simulink model "s1"  (R2022a)
settings: Solver=ode1  StartTime=0.0  StopTime=Tsin  FixedStep=0.01  RelTol=1e-3
values from neighbouring files (symbols this model uses):
  alpha1 = x1    [HHmododeslizante2.m]
  amp = 1    [HHmododeslizante2.m]
  beta1 = x2    [HHmododeslizante2.m]
  k5 = 0.3    [HHmododeslizante2.m]
  Lambda = x3    [HHmododeslizante2.m]
libraries: simulink x2
settings Model: Creator=L03037425  LastModifiedBy=danie
settings ModelReferenceCC: EnableRefExpFcnMdlSchedulingChecks=off
settings RTWCC: Description=Generic Real-Time Target

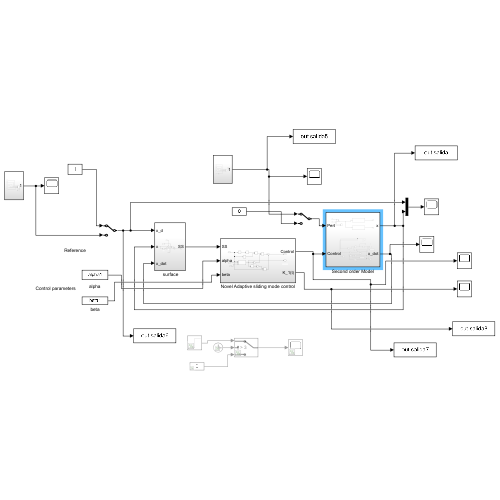
[thumbnail: Simulink's stored preview of the top-level diagram]
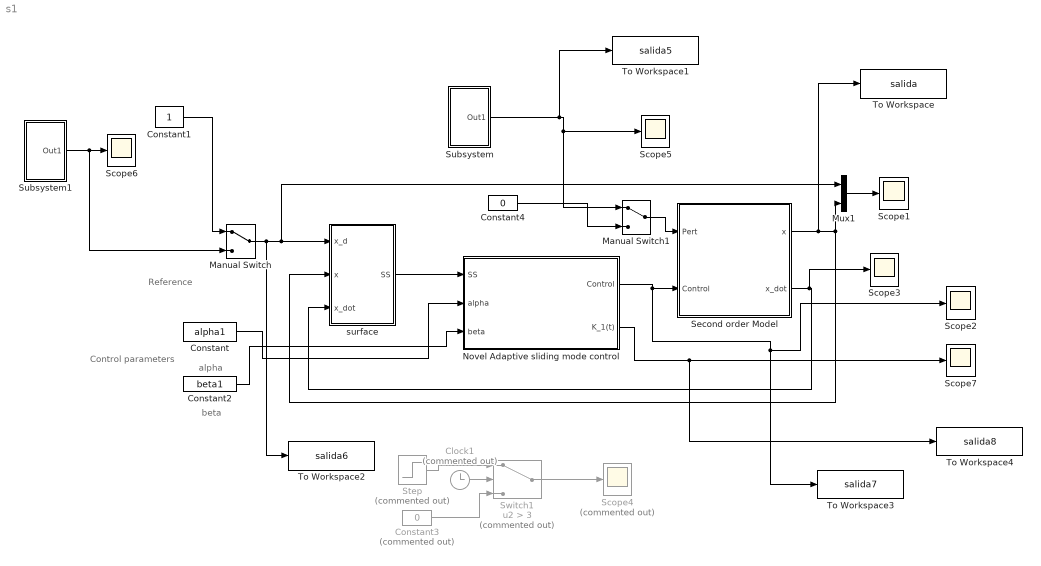
== system s1 ==
  note: Control parameters
  note: beta
  note: alpha
  note: Reference
  " surface" : Subsystem
  Clock1 : Clock  Commented=on
  Constant : Constant  Value=alpha1
  Constant1 : Constant
  Constant2 : Constant  Value=beta1
  Constant3 : Constant  Commented=on  Value=0
  Constant4 : Constant  Value=0
  Manual Switch : ManualSwitch
  Manual Switch1 : ManualSwitch
  Mux1 : Mux  Inputs=2
  Novel Adaptive sliding mode control : Subsystem
  Scope{1..3,5..7} (6 alike) : Scope
  Scope4 : Scope  Commented=on
  Second order Model : Subsystem
  Step : Step  Commented=on  Time=5  SampleTime=0
  Subsystem : Subsystem
  Subsystem1 : Subsystem
  Switch1 : Switch  Commented=on  Criteria=u2 > Threshold  Threshold=3  SaturateOnIntegerOverflow=off  InputSameDT=off
  To Workspace : ToWorkspace  VariableName=salida  SampleTime=-1
  To Workspace1 : ToWorkspace  VariableName=salida5  SampleTime=-1
  To Workspace2 : ToWorkspace  VariableName=salida6  SampleTime=-1
  To Workspace3 : ToWorkspace  VariableName=salida7  SampleTime=-1
  To Workspace4 : ToWorkspace  VariableName=salida8  SampleTime=-1
  wires:
  Constant1/1 -> Manual Switch/1
  " surface"/1(SS) -> Novel Adaptive sliding mode control/1(SS)
  Novel Adaptive sliding mode control/1(Control) -> To Workspace3/1, Scope2/1, Second order Model/2(Control)
  Manual Switch/1 -> To Workspace2/1, Mux1/1, " surface"/1(x_d)
  Second order Model/2(x_dot) -> Scope3/1, " surface"/3(x_dot)
  Second order Model/1(x) -> To Workspace/1, " surface"/2(x), Mux1/2
  Novel Adaptive sliding mode control/2(K_1(t)) -> To Workspace4/1, Scope7/1
  Constant/1 -> Novel Adaptive sliding mode control/2(alpha)
  Constant2/1 -> Novel Adaptive sliding mode control/3(beta)
  Mux1/1 -> Scope1/1
  Manual Switch1/1 -> Second order Model/1(Pert)
  Step/1 -> Switch1/1
  Switch1/1 -> Scope4/1
  Clock1/1 -> Switch1/2
  Constant3/1 -> Switch1/3
  Constant4/1 -> Manual Switch1/2
  Subsystem/1(Out1) -> To Workspace1/1, Manual Switch1/1, Scope5/1
  Subsystem1/1(Out1) -> Manual Switch/2, Scope6/1

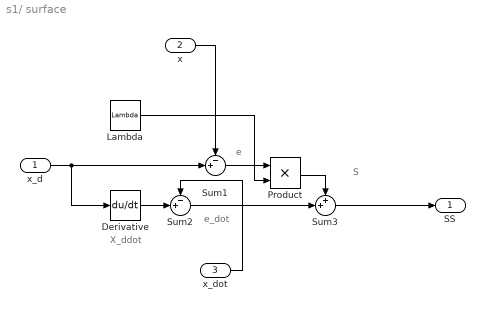
== system s1/ surface ==
  note: S
  note: e_dot
  note: e
  note: X_ddot
  x_d : Inport
  x : Inport  Port=2
  x_dot : Inport  Port=3
  Derivative : Derivative
  Lambda : Constant  Value=Lambda
  Product : Product
  Sum1 : Sum  Inputs=-+|
  Sum2 : Sum  Inputs=-+|
  Sum3 : Sum  Inputs=++|
  SS : Outport
  wires:
  Product/1 -> Sum3/1
  Sum2/1 -> Sum3/2
  x_d/1 -> Derivative/1, Sum1/2
  Lambda/1 -> Product/2
  Derivative/1 -> Sum2/2
  Sum1/1 -> Product/1
  Sum3/1 -> SS/1
  x/1 -> Sum1/1
  x_dot/1 -> Sum2/1

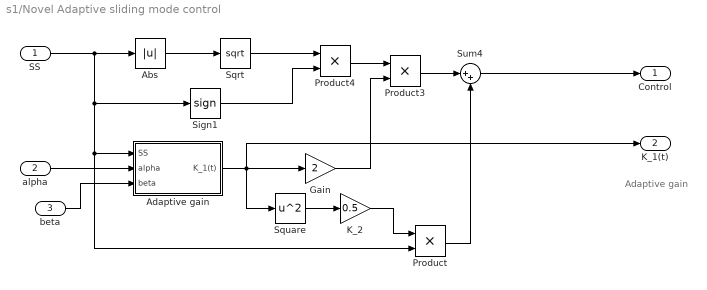
== system s1/Novel Adaptive sliding mode control ==
  note: Adaptive gain
  SS : Inport
  alpha : Inport  Port=2
  beta : Inport  Port=3
  Abs : Abs  SaturateOnIntegerOverflow=off
  Adaptive gain : Subsystem
  Gain : Gain  Gain=2
  K_2 : Gain  Gain=0.5
  Product : Product
  Product3 : Product
  Product4 : Product
  Sign1 : Signum
  Sqrt : Sqrt
  Square : Math  Operator=square
  Sum4 : Sum  Inputs=|++
  Control : Outport
  K_1(t) : Outport  Port=2
  wires:
  SS/1 -> Product/2, Adaptive gain/1(SS), Sign1/1, Abs/1
  Sqrt/1 -> Product4/1
  Product3/1 -> Sum4/1
  Abs/1 -> Sqrt/1
  Product4/1 -> Product3/1
  Sign1/1 -> Product4/2
  Sum4/1 -> Control/1
  Gain/1 -> Product3/2
  Adaptive gain/1(K_1(t)) -> K_1(t)/1, Gain/1, Square/1
  Product/1 -> Sum4/2
  K_2/1 -> Product/1
  Square/1 -> K_2/1
  alpha/1 -> Adaptive gain/2(alpha)
  beta/1 -> Adaptive gain/3(beta)

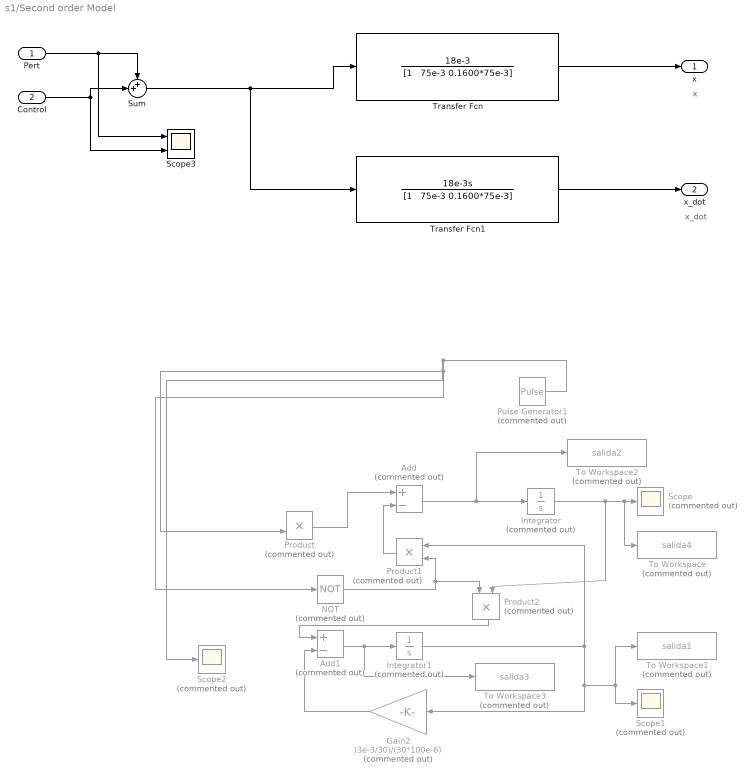
== system s1/Second order Model ==
  note: x
  note: x_dot
  Pert : Inport
  Control : Inport  Port=2
  Add : Sum  Commented=on  Inputs=+-
  Add1 : Sum  Commented=on  Inputs=+-
  Gain2 : Gain  Commented=on  Gain=(3e-3/30)/(30*100e-6)
  Integrator : Integrator  Commented=on
  Integrator1 : Integrator  Commented=on
  NOT : Logic  Commented=on  Operator=NOT  IconShape=distinctive  AllPortsSameDT=off  OutDataTypeStr=boolean
  Product : Product  Commented=on
  Product1 : Product  Commented=on
  Product2 : Product  Commented=on
  Pulse Generator1 : DiscretePulseGenerator  Commented=on  PulseType=Time based  Period=0.1  PulseWidth=0.6*100
  Scope : Scope  Commented=on
  Scope1 : Scope  Commented=on
  Scope2 : Scope  Commented=on
  Scope3 : Scope  NumInputPorts=2
  Sum : Sum  Inputs=++|
  To Workspace : ToWorkspace  Commented=on  VariableName=salida4  SampleTime=-1
  To Workspace1 : ToWorkspace  Commented=on  VariableName=salida1  SampleTime=-1
  To Workspace2 : ToWorkspace  Commented=on  VariableName=salida2  SampleTime=-1
  To Workspace3 : ToWorkspace  Commented=on  VariableName=salida3  SampleTime=-1
  Transfer Fcn : TransferFcn  Numerator=[18e-3]  Denominator="[1   75e-3 0.1600*75e-3]"
  Transfer Fcn1 : TransferFcn  Numerator=[18e-3 0]  Denominator="[1   75e-3 0.1600*75e-3]"
  x : Outport
  x_dot : Outport  Port=2
  wires:
  NOT/1 -> Product2/1, Product1/2
  Add1/1 -> Integrator1/1, To Workspace3/1
  Add/1 -> Integrator/1, To Workspace2/1
  Product1/1 -> Add/2
  Pulse Generator1/1 -> Scope2/1, Product/2, NOT/1
  Control/1 -> Sum/2, Scope3/2
  Product/1 -> Add/1
  Gain2/1 -> Add1/2
  Pert/1 -> Scope3/1, Sum/1
  Integrator1/1 -> Gain2/1, To Workspace1/1, Scope1/1, Product1/1
  Product2/1 -> Add1/1
  Integrator/1 -> To Workspace/1, Scope/1, Product2/2
  Sum/1 -> Transfer Fcn1/1, Transfer Fcn/1
  Transfer Fcn/1 -> x/1
  Transfer Fcn1/1 -> x_dot/1

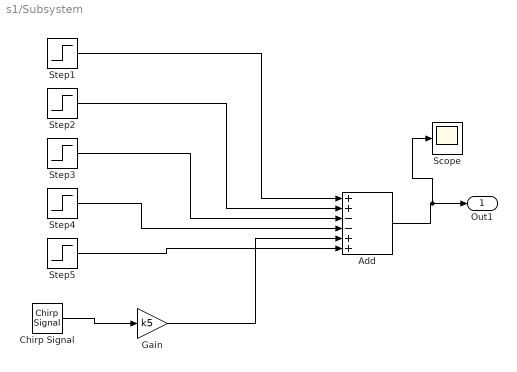
== system s1/Subsystem ==
  Add : Sum  Inputs=++--++
  Chirp Signal : simulink/Sources/Chirp Signal  f1=0.1  T=100  f2=10e3
  Gain : Gain  Gain=k5
  Scope : Scope
  Step1 : Step  Time=7  After=amp  SampleTime=0
  Step2 : Step  Time=9  After=amp  SampleTime=0
  Step3 : Step  Time=12  After=amp  SampleTime=0
  Step4 : Step  Time=25  After=amp  SampleTime=0
  Step5 : Step  Time=30  After=amp  SampleTime=0
  Out1 : Outport
  wires:
  Step2/1 -> Add/2
  Step4/1 -> Add/4
  Step1/1 -> Add/1
  Step3/1 -> Add/3
  Add/1 -> Scope/1, Out1/1
  Step5/1 -> Add/6
  Chirp Signal/1 -> Gain/1
  Gain/1 -> Add/5

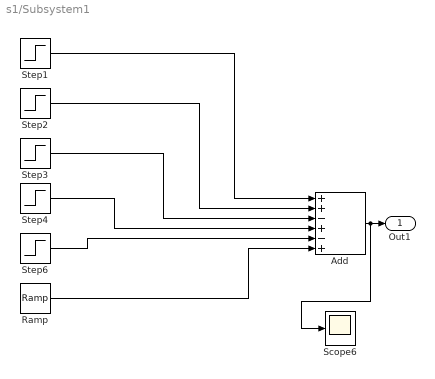
== system s1/Subsystem1 ==
  Add : Sum  Inputs=++-+-+
  Ramp : simulink/Sources/Ramp  slope=0.1  start=40  InitialOutput=0
  Scope6 : Scope
  Step1 : Step  Time=0  SampleTime=0
  Step2 : Step  Time=10  SampleTime=0
  Step3 : Step  Time=20  SampleTime=0
  Step4 : Step  Time=30  SampleTime=0
  Step6 : Step  Time=40  SampleTime=0
  Out1 : Outport
  wires:
  Step2/1 -> Add/2
  Step4/1 -> Add/4
  Step1/1 -> Add/1
  Step3/1 -> Add/3
  Add/1 -> Scope6/1, Out1/1
  Step6/1 -> Add/5
  Ramp/1 -> Add/6

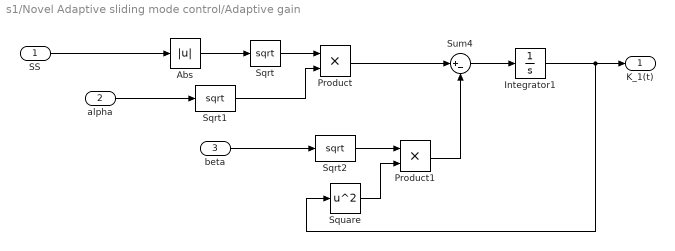
== system s1/Novel Adaptive sliding mode control/Adaptive gain ==
  SS : Inport
  alpha : Inport  Port=2
  beta : Inport  Port=3
  Abs : Abs  SaturateOnIntegerOverflow=off
  Integrator1 : Integrator  InitialCondition=0.1
  Product : Product
  Product1 : Product
  Sqrt : Sqrt
  Sqrt1 : Sqrt
  Sqrt2 : Sqrt
  Square : Math  Operator=square
  Sum4 : Sum  Inputs=|+-
  K_1(t) : Outport  VectorParamsAs1DForOutWhenUnconnected=off
  wires:
  Integrator1/1 -> Square/1, K_1(t)/1
  SS/1 -> Abs/1
  Sum4/1 -> Integrator1/1
  Abs/1 -> Sqrt/1
  Sqrt/1 -> Product/1
  Sqrt1/1 -> Product/2
  Product/1 -> Sum4/1
  beta/1 -> Sqrt2/1
  Sqrt2/1 -> Product1/1
  Square/1 -> Product1/2
  Product1/1 -> Sum4/2
  alpha/1 -> Sqrt1/1
